simulink model "simulated_motor"  (R2017a)
settings: Solver=FixedStepDiscrete  StartTime=0.0  StopTime=inf  FixedStep=0.001  RelTol=1e-3  EnableMultiTasking=on
values from neighbouring files (symbols this model uses):
  b = 3.5077e-06    [motor_params.mat]
  J = 3.2284e-06    [motor_params.mat]
  L = bwlabel(binimg)    [beginning_ip.m]    (also in motor_params.mat = 0.01; test_ip2.m)
  R = 4    [motor_params.mat]
undefined symbols (not defined in the file or in its folder): K
settings Model: SimulationMode=external  Creator=Venkatraman  LastModifiedBy=tbirdso
settings SolverCC: EnableConcurrentExecution=on
settings DataIOCC: LimitDataPoints=on  SaveFormat=Array  LoggingToFile=on
settings OptimizationCC: BlockReduction=off  OptimizeBlockIOStorage=off  BufferReuse=off  GlobalBufferReuse=off  ExpressionFolding=off  LocalBlockOutputs=off  LifeSpan=inf
settings DebuggingCC: SolverPrmCheckMsg=warning  SFUnexpectedBacktrackingDiag=warning  SFNoUnconditionalDefaultTransitionDiag=warning  SFExecutionAtInitializationDiag=none
settings HardwareCC: ProdBitPerPointer=32  ProdBitPerSizeT=32  ProdBitPerPtrDiffT=32  ProdLargestAtomicFloat=None  ProdWordSize=32  ProdLongLongMode=on  ProdHWDeviceType=Generic->32-bit x86 compatible  TargetBitPerPointer=64  TargetBitPerSizeT=64  TargetBitPerPtrDiffT=64  TargetLongLongMode=on  TargetIntDivRoundTo=Zero  TargetEndianess=LittleEndian  TargetWordSize=64  TargetHWDeviceType=MATLAB Host
settings ModelReferenceCC: PropagateSignalLabelsOutOfModel=off
settings RTWCC: SystemTargetFile=slrt.tlc  TemplateMakefile=slrt_default_tmf  Description=Simulink Real-Time  RTWVerbose=off  RTWCompilerOptimization=on
settings SimulinkRealTimeCC: GeneratePreprocessorConditionals=Disable all
settings ConfigComp: CovMetricSettings=dw  CovHtmlReporting=on  CovSaveCumulativeToWorkspaceVar=on  CovSaveSingleToWorkspaceVar=on  CovExternalEMLEnable=off  CovSFcnEnable=off

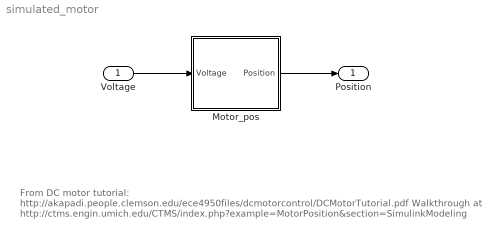
== system simulated_motor ==
  note: From DC motor tutorial: http://akapadi.people.clemson.edu/ece4950files/dcmotorcontrol/DCMotorTutorial.pdf
      |
      | Walkthrough at http://ctms.engin.umich.edu/CTMS/index.php?example=MotorPosition&section=SimulinkModeling
  Voltage : Inport
  Motor_pos : Subsystem
  Position : Outport
  wires:
  Voltage/1 -> Motor_pos/1(Voltage)
  Motor_pos/1(Position) -> Position/1

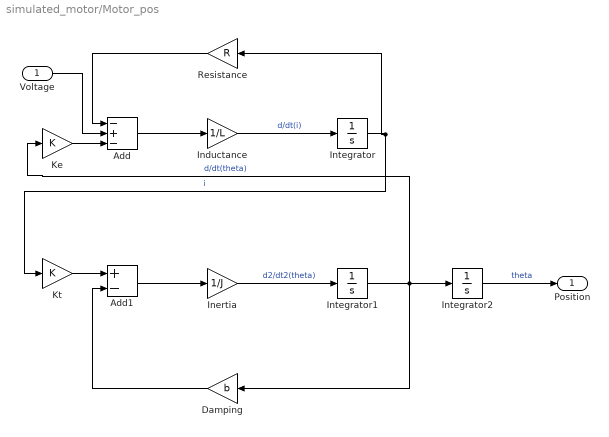
== system simulated_motor/Motor_pos ==
  Voltage : Inport
  Add : Sum  Inputs=-+-
  Add1 : Sum  Inputs=+-
  Damping : Gain  Gain=b
  Inductance : Gain  Gain=1/L
  "Inertia " : Gain  Gain=1/J
  Integrator : Integrator
  Integrator1 : Integrator
  Integrator2 : Integrator
  Ke : Gain  Gain=K
  Kt : Gain  Gain=K
  Resistance : Gain  Gain=R
  Position : Outport
  wires:
  Resistance/1 -> Add/1
  Ke/1 -> Add/3
  Kt/1 -> Add1/1
  Integrator/1 -> Resistance/1, Kt/1  "i"
  Add/1 -> Inductance/1
  Voltage/1 -> Add/2
  Integrator2/1 -> Position/1  "theta"
  Integrator1/1 -> Ke/1, Damping/1, Integrator2/1  "d/dt(theta)"
  Inductance/1 -> Integrator/1  "d/dt(i)"
  "Inertia "/1 -> Integrator1/1  "d2/dt2(theta)"
  Damping/1 -> Add1/2
  Add1/1 -> "Inertia "/1
